simulink model "Fuel_Pump_V3_1_20201113_20KHz"  (R2019b)
settings: configuration reference "Configuration" (kept outside this file)
PreLoadFcn:
  | RTWConfigurationCB('preloadfcn', bdroot);
values from neighbouring files (symbols this model uses):
  MotorPara_Base_Frq = 666.0    [fuel_pump_V3_1_20201113_20kHz.sldd]
  MotorPara_Base_I = 50.0    [fuel_pump_V3_1_20201113_20kHz.sldd]
  MotorPara_Base_RPM = 12000.0    [fuel_pump_V3_1_20201113_20kHz.sldd]
  MotorPara_Base_V = 28.0    [fuel_pump_V3_1_20201113_20kHz.sldd]
  MotorPara_Ld = 1.287E-5    [fuel_pump_V3_1_20201113_20kHz.sldd]
  MotorPara_Lq = 2.052E-5    [fuel_pump_V3_1_20201113_20kHz.sldd]
  MotorPara_Ls = 8.3475E-5    [fuel_pump_V3_1_20201113_20kHz.sldd]
  MotorPara_P = 4.0    [fuel_pump_V3_1_20201113_20kHz.sldd]
  MotorPara_Rs = 0.01638    [fuel_pump_V3_1_20201113_20kHz.sldd]
  TPBRD_HALF = 1875.0    [fuel_pump_V3_1_20201113_20kHz.sldd]
  Ts_1kHz = 0.001    [fuel_pump_V3_1_20201113_20kHz.sldd]
  Ts_200Hz = 0.005    [fuel_pump_V3_1_20201113_20kHz.sldd]
  Ts_20KHz = 5.0E-5    [fuel_pump_V3_1_20201113_20kHz.sldd]
  Ts_40Hz = 0.025    [fuel_pump_V3_1_20201113_20kHz.sldd]
  Ts_50Hz = 0.02    [fuel_pump_V3_1_20201113_20kHz.sldd]
undefined symbols (not defined in the file or in its folder): DiscIntNeverNeededParam, Down, Up
libraries: c280xlib x22, c2833xlib x6, c2837xDlib x4, c28xdmclib x4, etargetslib x4, dspstat3 x2, c2000lib x1, idelinklib_common x1
(part 1 of 4)
settings Model: DataDictionary=fuel_pump_V3_1_20201113_20kHz.sldd  ExtModeTrigDuration=8  OrderedModelArguments=off  Creator=Downstream  LastModifiedBy=Downstream
settings ConfigSetRef: SourceName=Configuration

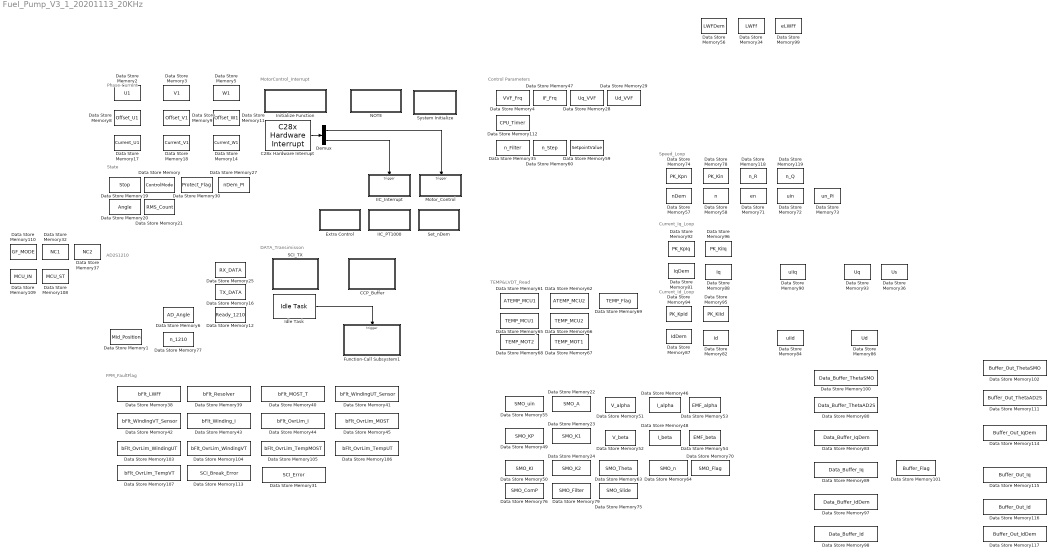
== system Fuel_Pump_V3_1_20201113_20KHz ==
  note: AD2S1210
  note: Phase-Current
  note: State
  note: DATA_Transimisson
  note: MotorControl_Interrupt
  note: Current_Id_Loop
  note: Current_Iq_Loop
  note: Control Parameters
  note: TEMP&LVDT_Read
  note: Speed_Loop
  note: FPM_FaultFlag
  C28x Hardware Interrupt : c2000lib/Scheduling/C28x Hardware Interrupt  irqnumbers=[1 8]  pienumbers=[6 1]  irqpriorities=[4 5]  irqpreempts=[0 0]  showinput=off  dspchiptype=C280X
      settings: SourceProductName=Embedded Coder Support Package for Texas Instruments C2000 Processors  SourceProductBaseCode=TIC2000
  CCP_Buffer : Subsystem  Priority=100  TreatAsAtomicUnit=on  SystemSampleTime=Ts_200Hz
  Data Store Memory : DataStoreMemory  DataStoreName=ControlMode  ReadBeforeWriteMsg=warning  WriteAfterWriteMsg=warning  WriteAfterReadMsg=warning  InitialValue=4  ShowAdditionalParam=off  OutDataTypeStr=uint16
      settings: RTWStateStorageClass=ExportedGlobal
  Data Store Memory1 : DataStoreMemory  DataStoreName=Mid_Position  ReadBeforeWriteMsg=warning  WriteAfterWriteMsg=warning  WriteAfterReadMsg=warning  ShowAdditionalParam=off  OutDataTypeStr=uint16
      settings: RTWStateStorageClass=ExportedGlobal
  Data Store Memory100 : DataStoreMemory  DataStoreName=Data_Buffer_ThetaSMO  ReadBeforeWriteMsg=warning  WriteAfterWriteMsg=warning  WriteAfterReadMsg=warning  InitialValue=zeros(1,1000)  ShowAdditionalParam=off  OutDataTypeStr=single
      settings: RTWStateStorageClass=ExportedGlobal
  Data Store Memory101 : DataStoreMemory  DataStoreName=Buffer_Flag  ReadBeforeWriteMsg=warning  WriteAfterWriteMsg=warning  WriteAfterReadMsg=warning  ShowAdditionalParam=off  OutDataTypeStr=uint16
      settings: RTWStateStorageClass=ExportedGlobal
  Data Store Memory102 : DataStoreMemory  DataStoreName=Buffer_Out_ThetaSMO  ReadBeforeWriteMsg=warning  WriteAfterWriteMsg=warning  WriteAfterReadMsg=warning  ShowAdditionalParam=off  OutDataTypeStr=single
      settings: RTWStateStorageClass=ExportedGlobal
  Data Store Memory103 : DataStoreMemory  DataStoreName=bFlt_OvrLim_WindingUT  ReadBeforeWriteMsg=warning  WriteAfterWriteMsg=warning  WriteAfterReadMsg=warning  ShowAdditionalParam=off  OutDataTypeStr=uint16
      settings: RTWStateStorageClass=ExportedGlobal
  Data Store Memory104 : DataStoreMemory  DataStoreName=bFlt_OvrLim_WindingVT  ReadBeforeWriteMsg=warning  WriteAfterWriteMsg=warning  WriteAfterReadMsg=warning  ShowAdditionalParam=off  OutDataTypeStr=uint16
      settings: RTWStateStorageClass=ExportedGlobal
  Data Store Memory105 : DataStoreMemory  DataStoreName=bFlt_OvrLim_TempMOST  ReadBeforeWriteMsg=warning  WriteAfterWriteMsg=warning  WriteAfterReadMsg=warning  ShowAdditionalParam=off  OutDataTypeStr=uint16
      settings: RTWStateStorageClass=ExportedGlobal
  Data Store Memory106 : DataStoreMemory  DataStoreName=bFlt_OvrLim_TempUT  ReadBeforeWriteMsg=warning  WriteAfterWriteMsg=warning  WriteAfterReadMsg=warning  ShowAdditionalParam=off  OutDataTypeStr=uint16
      settings: RTWStateStorageClass=ExportedGlobal
  Data Store Memory107 : DataStoreMemory  DataStoreName=bFlt_OvrLim_TempVT  ReadBeforeWriteMsg=warning  WriteAfterWriteMsg=warning  WriteAfterReadMsg=warning  ShowAdditionalParam=off  OutDataTypeStr=uint16
      settings: RTWStateStorageClass=ExportedGlobal
  Data Store Memory108 : DataStoreMemory  DataStoreName=MCU_ST  ReadBeforeWriteMsg=warning  WriteAfterWriteMsg=warning  WriteAfterReadMsg=warning  ShowAdditionalParam=off  OutDataTypeStr=uint16
      settings: RTWStateStorageClass=ExportedGlobal
  Data Store Memory109 : DataStoreMemory  DataStoreName=MCU_IN  ReadBeforeWriteMsg=warning  WriteAfterWriteMsg=warning  WriteAfterReadMsg=warning  ShowAdditionalParam=off  OutDataTypeStr=uint16
      settings: RTWStateStorageClass=ExportedGlobal
  Data Store Memory11 : DataStoreMemory  DataStoreName=Offset_W1  ReadBeforeWriteMsg=warning  WriteAfterWriteMsg=warning  WriteAfterReadMsg=warning  ShowAdditionalParam=off  OutDataTypeStr=uint16
      settings: RTWStateStorageClass=ExportedGlobal
  Data Store Memory110 : DataStoreMemory  DataStoreName=GF_MODE  ReadBeforeWriteMsg=warning  WriteAfterWriteMsg=warning  WriteAfterReadMsg=warning  ShowAdditionalParam=off  OutDataTypeStr=uint16
      settings: RTWStateStorageClass=ExportedGlobal
  Data Store Memory111 : DataStoreMemory  DataStoreName=Buffer_Out_ThetaAD2S  ReadBeforeWriteMsg=warning  WriteAfterWriteMsg=warning  WriteAfterReadMsg=warning  ShowAdditionalParam=off  OutDataTypeStr=single
      settings: RTWStateStorageClass=ExportedGlobal
  Data Store Memory112 : DataStoreMemory  DataStoreName=CPU_Timer  ReadBeforeWriteMsg=warning  WriteAfterWriteMsg=warning  WriteAfterReadMsg=warning  ShowAdditionalParam=off  OutDataTypeStr=uint32
      settings: RTWStateStorageClass=ExportedGlobal
  Data Store Memory113 : DataStoreMemory  DataStoreName=SCI_Break_Error  ReadBeforeWriteMsg=warning  WriteAfterWriteMsg=warning  WriteAfterReadMsg=warning  ShowAdditionalParam=off  OutDataTypeStr=uint16
      settings: RTWStateStorageClass=ExportedGlobal
  Data Store Memory114 : DataStoreMemory  DataStoreName=Buffer_Out_IqDem  ReadBeforeWriteMsg=warning  WriteAfterWriteMsg=warning  WriteAfterReadMsg=warning  ShowAdditionalParam=off  OutDataTypeStr=single
      settings: RTWStateStorageClass=ExportedGlobal
  Data Store Memory115 : DataStoreMemory  DataStoreName=Buffer_Out_Iq  ReadBeforeWriteMsg=warning  WriteAfterWriteMsg=warning  WriteAfterReadMsg=warning  ShowAdditionalParam=off  OutDataTypeStr=single
      settings: RTWStateStorageClass=ExportedGlobal
  Data Store Memory116 : DataStoreMemory  DataStoreName=Buffer_Out_Id  ReadBeforeWriteMsg=warning  WriteAfterWriteMsg=warning  WriteAfterReadMsg=warning  ShowAdditionalParam=off  OutDataTypeStr=single
      settings: RTWStateStorageClass=ExportedGlobal
  Data Store Memory117 : DataStoreMemory  DataStoreName=Buffer_Out_IdDem  ReadBeforeWriteMsg=warning  WriteAfterWriteMsg=warning  WriteAfterReadMsg=warning  ShowAdditionalParam=off  OutDataTypeStr=single
      settings: RTWStateStorageClass=ExportedGlobal
  Data Store Memory118 : DataStoreMemory  DataStoreName=n_R  ReadBeforeWriteMsg=warning  WriteAfterWriteMsg=warning  WriteAfterReadMsg=warning  ShowAdditionalParam=off  OutDataTypeStr=single
      settings: RTWStateStorageClass=ExportedGlobal
  Data Store Memory119 : DataStoreMemory  DataStoreName=n_Q  ReadBeforeWriteMsg=warning  WriteAfterWriteMsg=warning  WriteAfterReadMsg=warning  ShowAdditionalParam=off  OutDataTypeStr=single
      settings: RTWStateStorageClass=ExportedGlobal
  Data Store Memory12 : DataStoreMemory  DataStoreName=Ready_1210  ReadBeforeWriteMsg=warning  WriteAfterWriteMsg=warning  WriteAfterReadMsg=warning  ShowAdditionalParam=off  OutDataTypeStr=single
      settings: RTWStateStorageClass=ExportedGlobal
  Data Store Memory14 : DataStoreMemory  DataStoreName=Current_W1  ReadBeforeWriteMsg=warning  WriteAfterWriteMsg=warning  WriteAfterReadMsg=warning  ShowAdditionalParam=off  OutDataTypeStr=single
      settings: RTWStateStorageClass=ExportedGlobal
  Data Store Memory16 : DataStoreMemory  DataStoreName=TX_DATA  ReadBeforeWriteMsg=warning  WriteAfterWriteMsg=warning  WriteAfterReadMsg=warning  ShowAdditionalParam=off  OutDataTypeStr=uint16
      settings: RTWStateStorageClass=ExportedGlobal
  Data Store Memory17 : DataStoreMemory  DataStoreName=Current_U1  ReadBeforeWriteMsg=warning  WriteAfterWriteMsg=warning  WriteAfterReadMsg=warning  ShowAdditionalParam=off  OutDataTypeStr=single
      settings: RTWStateStorageClass=ExportedGlobal
  Data Store Memory18 : DataStoreMemory  DataStoreName=Current_V1  ReadBeforeWriteMsg=warning  WriteAfterWriteMsg=warning  WriteAfterReadMsg=warning  ShowAdditionalParam=off  OutDataTypeStr=single
      settings: RTWStateStorageClass=ExportedGlobal
  Data Store Memory19 : DataStoreMemory  DataStoreName=Stop  ReadBeforeWriteMsg=warning  WriteAfterWriteMsg=warning  WriteAfterReadMsg=warning  ShowAdditionalParam=off  OutDataTypeStr=uint16
      settings: RTWStateStorageClass=ExportedGlobal
  Data Store Memory2 : DataStoreMemory  DataStoreName=U1  ReadBeforeWriteMsg=warning  WriteAfterWriteMsg=warning  WriteAfterReadMsg=warning  ShowAdditionalParam=off  OutDataTypeStr=uint16
      settings: RTWStateStorageClass=ExportedGlobal
  Data Store Memory20 : DataStoreMemory  DataStoreName=Angle  ReadBeforeWriteMsg=warning  WriteAfterWriteMsg=warning  WriteAfterReadMsg=warning  ShowAdditionalParam=off  OutDataTypeStr=single
      settings: RTWStateStorageClass=ExportedGlobal
  Data Store Memory21 : DataStoreMemory  DataStoreName=RMS_Count  ReadBeforeWriteMsg=warning  WriteAfterWriteMsg=warning  WriteAfterReadMsg=warning  ShowAdditionalParam=off  OutDataTypeStr=uint16
      settings: RTWStateStorageClass=ExportedGlobal
  Data Store Memory22 : DataStoreMemory  DataStoreName=SMO_A  ReadBeforeWriteMsg=warning  WriteAfterWriteMsg=warning  WriteAfterReadMsg=warning  ShowAdditionalParam=off  OutDataTypeStr=single
      settings: RTWStateStorageClass=ExportedGlobal
  Data Store Memory23 : DataStoreMemory  DataStoreName=SMO_K1  ReadBeforeWriteMsg=warning  WriteAfterWriteMsg=warning  WriteAfterReadMsg=warning  ShowAdditionalParam=off  OutDataTypeStr=single
      settings: RTWStateStorageClass=ExportedGlobal
  Data Store Memory24 : DataStoreMemory  DataStoreName=SMO_K2  ReadBeforeWriteMsg=warning  WriteAfterWriteMsg=warning  WriteAfterReadMsg=warning  ShowAdditionalParam=off  OutDataTypeStr=single
      settings: RTWStateStorageClass=ExportedGlobal
  Data Store Memory25 : DataStoreMemory  DataStoreName=RX_DATA  ReadBeforeWriteMsg=warning  WriteAfterWriteMsg=warning  WriteAfterReadMsg=warning  ShowAdditionalParam=off  OutDataTypeStr=uint16
      settings: RTWStateStorageClass=ExportedGlobal
  Data Store Memory27 : DataStoreMemory  DataStoreName=nDem_PI  ReadBeforeWriteMsg=warning  WriteAfterWriteMsg=warning  WriteAfterReadMsg=warning  ShowAdditionalParam=off  OutDataTypeStr=single
      settings: RTWStateStorageClass=ExportedGlobal
  Data Store Memory28 : DataStoreMemory  DataStoreName=Uq_VVF  ReadBeforeWriteMsg=warning  WriteAfterWriteMsg=warning  WriteAfterReadMsg=warning  ShowAdditionalParam=off  OutDataTypeStr=single
      settings: RTWStateStorageClass=ExportedGlobal
  Data Store Memory29 : DataStoreMemory  DataStoreName=Ud_VVF  ReadBeforeWriteMsg=warning  WriteAfterWriteMsg=warning  WriteAfterReadMsg=warning  ShowAdditionalParam=off  OutDataTypeStr=single
      settings: RTWStateStorageClass=ExportedGlobal
  Data Store Memory3 : DataStoreMemory  DataStoreName=V1  ReadBeforeWriteMsg=warning  WriteAfterWriteMsg=warning  WriteAfterReadMsg=warning  ShowAdditionalParam=off  OutDataTypeStr=uint16
      settings: RTWStateStorageClass=ExportedGlobal
  Data Store Memory30 : DataStoreMemory  DataStoreName=Protect_Flag  ReadBeforeWriteMsg=warning  WriteAfterWriteMsg=warning  WriteAfterReadMsg=warning  ShowAdditionalParam=off  OutDataTypeStr=uint16
      settings: RTWStateStorageClass=ExportedGlobal
  Data Store Memory31 : DataStoreMemory  DataStoreName=SCI_Error  ReadBeforeWriteMsg=warning  WriteAfterWriteMsg=warning  WriteAfterReadMsg=warning  ShowAdditionalParam=off  OutDataTypeStr=uint16
      settings: RTWStateStorageClass=ExportedGlobal
  Data Store Memory32 : DataStoreMemory  DataStoreName=NC1  ReadBeforeWriteMsg=warning  WriteAfterWriteMsg=warning  WriteAfterReadMsg=warning  ShowAdditionalParam=off  OutDataTypeStr=uint16
      settings: RTWStateStorageClass=ExportedGlobal
  Data Store Memory34 : DataStoreMemory  DataStoreName=LWFf  ReadBeforeWriteMsg=warning  WriteAfterWriteMsg=warning  WriteAfterReadMsg=warning  ShowAdditionalParam=off  OutDataTypeStr=single
      settings: RTWStateStorageClass=ExportedGlobal
  Data Store Memory35 : DataStoreMemory  DataStoreName=n_Filter  ReadBeforeWriteMsg=warning  WriteAfterWriteMsg=warning  WriteAfterReadMsg=warning  InitialValue=2000  ShowAdditionalParam=off  OutDataTypeStr=single
      settings: RTWStateStorageClass=ExportedGlobal
  Data Store Memory36 : DataStoreMemory  DataStoreName=Us  ReadBeforeWriteMsg=warning  WriteAfterWriteMsg=warning  WriteAfterReadMsg=warning  ShowAdditionalParam=off  OutDataTypeStr=single
      settings: RTWStateStorageClass=ExportedGlobal
  Data Store Memory37 : DataStoreMemory  DataStoreName=NC2  ReadBeforeWriteMsg=warning  WriteAfterWriteMsg=warning  WriteAfterReadMsg=warning  ShowAdditionalParam=off  OutDataTypeStr=uint16
      settings: RTWStateStorageClass=ExportedGlobal
  Data Store Memory38 : DataStoreMemory  DataStoreName=bFlt_LWFf  ReadBeforeWriteMsg=warning  WriteAfterWriteMsg=warning  WriteAfterReadMsg=warning  ShowAdditionalParam=off  OutDataTypeStr=uint16
      settings: RTWStateStorageClass=ExportedGlobal
  Data Store Memory39 : DataStoreMemory  DataStoreName=bFlt_Resolver  ReadBeforeWriteMsg=warning  WriteAfterWriteMsg=warning  WriteAfterReadMsg=warning  ShowAdditionalParam=off  OutDataTypeStr=uint16
      settings: RTWStateStorageClass=ExportedGlobal
  Data Store Memory4 : DataStoreMemory  DataStoreName=VVF_Frq  ReadBeforeWriteMsg=warning  WriteAfterWriteMsg=warning  WriteAfterReadMsg=warning  ShowAdditionalParam=off  OutDataTypeStr=fixdt(1,32,29)
      settings: RTWStateStorageClass=ExportedGlobal
  Data Store Memory40 : DataStoreMemory  DataStoreName=bFlt_MOST_T  ReadBeforeWriteMsg=warning  WriteAfterWriteMsg=warning  WriteAfterReadMsg=warning  ShowAdditionalParam=off  OutDataTypeStr=uint16
      settings: RTWStateStorageClass=ExportedGlobal
  Data Store Memory41 : DataStoreMemory  DataStoreName=bFlt_WindingUT_Sensor  ReadBeforeWriteMsg=warning  WriteAfterWriteMsg=warning  WriteAfterReadMsg=warning  ShowAdditionalParam=off  OutDataTypeStr=uint16
      settings: RTWStateStorageClass=ExportedGlobal
  Data Store Memory42 : DataStoreMemory  DataStoreName=bFlt_WindingVT_Sensor  ReadBeforeWriteMsg=warning  WriteAfterWriteMsg=warning  WriteAfterReadMsg=warning  ShowAdditionalParam=off  OutDataTypeStr=uint16
      settings: RTWStateStorageClass=ExportedGlobal
  Data Store Memory43 : DataStoreMemory  DataStoreName=bFlt_Winding_I  ReadBeforeWriteMsg=warning  WriteAfterWriteMsg=warning  WriteAfterReadMsg=warning  ShowAdditionalParam=off  OutDataTypeStr=uint16
      settings: RTWStateStorageClass=ExportedGlobal
  Data Store Memory44 : DataStoreMemory  DataStoreName=bFlt_OvrLim_I  ReadBeforeWriteMsg=warning  WriteAfterWriteMsg=warning  WriteAfterReadMsg=warning  ShowAdditionalParam=off  OutDataTypeStr=uint16
      settings: RTWStateStorageClass=ExportedGlobal
  Data Store Memory45 : DataStoreMemory  DataStoreName=bFlt_OvrLim_MOST  ReadBeforeWriteMsg=warning  WriteAfterWriteMsg=warning  WriteAfterReadMsg=warning  ShowAdditionalParam=off  OutDataTypeStr=uint16
      settings: RTWStateStorageClass=ExportedGlobal
  Data Store Memory46 : DataStoreMemory  DataStoreName=I_alpha  ReadBeforeWriteMsg=warning  WriteAfterWriteMsg=warning  WriteAfterReadMsg=warning  ShowAdditionalParam=off  OutDataTypeStr=single
      settings: RTWStateStorageClass=ExportedGlobal
  Data Store Memory47 : DataStoreMemory  DataStoreName=IF_Frq  ReadBeforeWriteMsg=warning  WriteAfterWriteMsg=warning  WriteAfterReadMsg=warning  ShowAdditionalParam=off  OutDataTypeStr=fixdt(1,32,29)
      settings: RTWStateStorageClass=ExportedGlobal
  Data Store Memory48 : DataStoreMemory  DataStoreName=I_beta  ReadBeforeWriteMsg=warning  WriteAfterWriteMsg=warning  WriteAfterReadMsg=warning  ShowAdditionalParam=off  OutDataTypeStr=single
      settings: RTWStateStorageClass=ExportedGlobal
  Data Store Memory49 : DataStoreMemory  DataStoreName=SMO_KP  ReadBeforeWriteMsg=warning  WriteAfterWriteMsg=warning  WriteAfterReadMsg=warning  ShowAdditionalParam=off  OutDataTypeStr=single
      settings: RTWStateStorageClass=ExportedGlobal
  Data Store Memory5 : DataStoreMemory  DataStoreName=W1  ReadBeforeWriteMsg=warning  WriteAfterWriteMsg=warning  WriteAfterReadMsg=warning  ShowAdditionalParam=off  OutDataTypeStr=uint16
      settings: RTWStateStorageClass=ExportedGlobal
  Data Store Memory50 : DataStoreMemory  DataStoreName=SMO_KI  ReadBeforeWriteMsg=warning  WriteAfterWriteMsg=warning  WriteAfterReadMsg=warning  ShowAdditionalParam=off  OutDataTypeStr=single
      settings: RTWStateStorageClass=ExportedGlobal
  Data Store Memory51 : DataStoreMemory  DataStoreName=V_alpha  ReadBeforeWriteMsg=warning  WriteAfterWriteMsg=warning  WriteAfterReadMsg=warning  ShowAdditionalParam=off  OutDataTypeStr=single
      settings: RTWStateStorageClass=ExportedGlobal
  Data Store Memory52 : DataStoreMemory  DataStoreName=V_beta  ReadBeforeWriteMsg=warning  WriteAfterWriteMsg=warning  WriteAfterReadMsg=warning  ShowAdditionalParam=off  OutDataTypeStr=single
      settings: RTWStateStorageClass=ExportedGlobal
  Data Store Memory53 : DataStoreMemory  DataStoreName=EMF_alpha  ReadBeforeWriteMsg=warning  WriteAfterWriteMsg=warning  WriteAfterReadMsg=warning  ShowAdditionalParam=off  OutDataTypeStr=single
      settings: RTWStateStorageClass=ExportedGlobal
  Data Store Memory54 : DataStoreMemory  DataStoreName=EMF_beta  ReadBeforeWriteMsg=warning  WriteAfterWriteMsg=warning  WriteAfterReadMsg=warning  ShowAdditionalParam=off  OutDataTypeStr=single
      settings: RTWStateStorageClass=ExportedGlobal
  Data Store Memory55 : DataStoreMemory  DataStoreName=SMO_uin  ReadBeforeWriteMsg=warning  WriteAfterWriteMsg=warning  WriteAfterReadMsg=warning  ShowAdditionalParam=off  OutDataTypeStr=single
      settings: RTWStateStorageClass=ExportedGlobal
  Data Store Memory56 : DataStoreMemory  DataStoreName=LWFDem  ReadBeforeWriteMsg=warning  WriteAfterWriteMsg=warning  WriteAfterReadMsg=warning  ShowAdditionalParam=off  OutDataTypeStr=single
      settings: RTWStateStorageClass=ExportedGlobal
  Data Store Memory57 : DataStoreMemory  DataStoreName=nDem  ReadBeforeWriteMsg=warning  WriteAfterWriteMsg=warning  WriteAfterReadMsg=warning  ShowAdditionalParam=off  OutDataTypeStr=single
      settings: RTWStateStorageClass=ExportedGlobal
  Data Store Memory58 : DataStoreMemory  DataStoreName=n  ReadBeforeWriteMsg=warning  WriteAfterWriteMsg=warning  WriteAfterReadMsg=warning  ShowAdditionalParam=off  OutDataTypeStr=single
      settings: RTWStateStorageClass=ExportedGlobal
  Data Store Memory59 : DataStoreMemory  DataStoreName=SetpointValue  ReadBeforeWriteMsg=warning  WriteAfterWriteMsg=warning  WriteAfterReadMsg=warning  ShowAdditionalParam=off  OutDataTypeStr=single
      settings: RTWStateStorageClass=ExportedGlobal
  Data Store Memory6 : DataStoreMemory  DataStoreName=AD_Angle  ReadBeforeWriteMsg=warning  WriteAfterWriteMsg=warning  WriteAfterReadMsg=warning  ShowAdditionalParam=off  OutDataTypeStr=single
      settings: RTWStateStorageClass=ExportedGlobal
  Data Store Memory60 : DataStoreMemory  DataStoreName=n_Step  ReadBeforeWriteMsg=warning  WriteAfterWriteMsg=warning  WriteAfterReadMsg=warning  InitialValue=5/15000  ShowAdditionalParam=off  OutDataTypeStr=single
      settings: RTWStateStorageClass=ExportedGlobal
  Data Store Memory61 : DataStoreMemory  DataStoreName=ATEMP_MCU1  ReadBeforeWriteMsg=warning  WriteAfterWriteMsg=warning  WriteAfterReadMsg=warning  ShowAdditionalParam=off  OutDataTypeStr=uint16
      settings: RTWStateStorageClass=ExportedGlobal
  Data Store Memory62 : DataStoreMemory  DataStoreName=ATEMP_MCU2  ReadBeforeWriteMsg=warning  WriteAfterWriteMsg=warning  WriteAfterReadMsg=warning  ShowAdditionalParam=off  OutDataTypeStr=uint16
      settings: RTWStateStorageClass=ExportedGlobal
  Data Store Memory63 : DataStoreMemory  DataStoreName=SMO_Theta  ReadBeforeWriteMsg=warning  WriteAfterWriteMsg=warning  WriteAfterReadMsg=warning  ShowAdditionalParam=off  OutDataTypeStr=single
      settings: RTWStateStorageClass=ExportedGlobal
  Data Store Memory64 : DataStoreMemory  DataStoreName=SMO_n  ReadBeforeWriteMsg=warning  WriteAfterWriteMsg=warning  WriteAfterReadMsg=warning  ShowAdditionalParam=off  OutDataTypeStr=single
      settings: RTWStateStorageClass=ExportedGlobal
  Data Store Memory65 : DataStoreMemory  DataStoreName=TEMP_MCU1  ReadBeforeWriteMsg=warning  WriteAfterWriteMsg=warning  WriteAfterReadMsg=warning  ShowAdditionalParam=off  OutDataTypeStr=single
      settings: RTWStateStorageClass=ExportedGlobal
  Data Store Memory66 : DataStoreMemory  DataStoreName=TEMP_MCU2  ReadBeforeWriteMsg=warning  WriteAfterWriteMsg=warning  WriteAfterReadMsg=warning  ShowAdditionalParam=off  OutDataTypeStr=single
      settings: RTWStateStorageClass=ExportedGlobal
  Data Store Memory67 : DataStoreMemory  DataStoreName=TEMP_MOT1  ReadBeforeWriteMsg=warning  WriteAfterWriteMsg=warning  WriteAfterReadMsg=warning  ShowAdditionalParam=off  OutDataTypeStr=single
      settings: RTWStateStorageClass=ExportedGlobal
  Data Store Memory68 : DataStoreMemory  DataStoreName=TEMP_MOT2  ReadBeforeWriteMsg=warning  WriteAfterWriteMsg=warning  WriteAfterReadMsg=warning  ShowAdditionalParam=off  OutDataTypeStr=single
      settings: RTWStateStorageClass=ExportedGlobal
  Data Store Memory69 : DataStoreMemory  DataStoreName=TEMP_Flag  ReadBeforeWriteMsg=warning  WriteAfterWriteMsg=warning  WriteAfterReadMsg=warning  ShowAdditionalParam=off  OutDataTypeStr=uint16
      settings: RTWStateStorageClass=ExportedGlobal
  Data Store Memory70 : DataStoreMemory  DataStoreName=SMO_Flag  ReadBeforeWriteMsg=warning  WriteAfterWriteMsg=warning  WriteAfterReadMsg=warning  ShowAdditionalParam=off  OutDataTypeStr=uint16
      settings: RTWStateStorageClass=ExportedGlobal
  Data Store Memory71 : DataStoreMemory  DataStoreName=en  ReadBeforeWriteMsg=warning  WriteAfterWriteMsg=warning  WriteAfterReadMsg=warning  ShowAdditionalParam=off  OutDataTypeStr=single
      settings: RTWStateStorageClass=ExportedGlobal
  Data Store Memory72 : DataStoreMemory  DataStoreName=uin  ReadBeforeWriteMsg=warning  WriteAfterWriteMsg=warning  WriteAfterReadMsg=warning  ShowAdditionalParam=off  OutDataTypeStr=single
      settings: RTWStateStorageClass=ExportedGlobal
  Data Store Memory73 : DataStoreMemory  DataStoreName=un_PI  ReadBeforeWriteMsg=warning  WriteAfterWriteMsg=warning  WriteAfterReadMsg=warning  ShowAdditionalParam=off  OutDataTypeStr=single
      settings: RTWStateStorageClass=ExportedGlobal
  Data Store Memory74 : DataStoreMemory  DataStoreName=PK_Kpn  ReadBeforeWriteMsg=warning  WriteAfterWriteMsg=warning  WriteAfterReadMsg=warning  ShowAdditionalParam=off  OutDataTypeStr=single
      settings: RTWStateStorageClass=ExportedGlobal
  Data Store Memory75 : DataStoreMemory  DataStoreName=SMO_Slide  ReadBeforeWriteMsg=warning  WriteAfterWriteMsg=warning  WriteAfterReadMsg=warning  ShowAdditionalParam=off  OutDataTypeStr=single
      settings: RTWStateStorageClass=ExportedGlobal
  Data Store Memory76 : DataStoreMemory  DataStoreName=SMO_ComP  ReadBeforeWriteMsg=warning  WriteAfterWriteMsg=warning  WriteAfterReadMsg=warning  ShowAdditionalParam=off  OutDataTypeStr=single
      settings: RTWStateStorageClass=ExportedGlobal
  Data Store Memory77 : DataStoreMemory  DataStoreName=n_1210  ReadBeforeWriteMsg=warning  WriteAfterWriteMsg=warning  WriteAfterReadMsg=warning  ShowAdditionalParam=off  OutDataTypeStr=single
      settings: RTWStateStorageClass=ExportedGlobal
  Data Store Memory78 : DataStoreMemory  DataStoreName=PK_Kin  ReadBeforeWriteMsg=warning  WriteAfterWriteMsg=warning  WriteAfterReadMsg=warning  ShowAdditionalParam=off  OutDataTypeStr=single
      settings: RTWStateStorageClass=ExportedGlobal
  Data Store Memory79 : DataStoreMemory  DataStoreName=SMO_Filter  ReadBeforeWriteMsg=warning  WriteAfterWriteMsg=warning  WriteAfterReadMsg=warning  ShowAdditionalParam=off  OutDataTypeStr=single
      settings: RTWStateStorageClass=ExportedGlobal
  Data Store Memory8 : DataStoreMemory  DataStoreName=Offset_U1  ReadBeforeWriteMsg=warning  WriteAfterWriteMsg=warning  WriteAfterReadMsg=warning  ShowAdditionalParam=off  OutDataTypeStr=uint16
      settings: RTWStateStorageClass=ExportedGlobal
  Data Store Memory80 : DataStoreMemory  DataStoreName=Data_Buffer_ThetaAD2S  ReadBeforeWriteMsg=warning  WriteAfterWriteMsg=warning  WriteAfterReadMsg=warning  InitialValue=zeros(1,1000)  ShowAdditionalParam=off  OutDataTypeStr=single
      settings: RTWStateStorageClass=ExportedGlobal
  Data Store Memory81 : DataStoreMemory  DataStoreName=IqDem  ReadBeforeWriteMsg=warning  WriteAfterWriteMsg=warning  WriteAfterReadMsg=warning  ShowAdditionalParam=off  OutDataTypeStr=single
      settings: RTWStateStorageClass=ExportedGlobal
  Data Store Memory82 : DataStoreMemory  DataStoreName=Id  ReadBeforeWriteMsg=warning  WriteAfterWriteMsg=warning  WriteAfterReadMsg=warning  ShowAdditionalParam=off  OutDataTypeStr=single
      settings: RTWStateStorageClass=ExportedGlobal
  Data Store Memory83 : DataStoreMemory  DataStoreName=Data_Buffer_IqDem  ReadBeforeWriteMsg=warning  WriteAfterWriteMsg=warning  WriteAfterReadMsg=warning  InitialValue=zeros(1,1000)  ShowAdditionalParam=off  OutDataTypeStr=single
      settings: RTWStateStorageClass=ExportedGlobal
  Data Store Memory84 : DataStoreMemory  DataStoreName=uiId  ReadBeforeWriteMsg=warning  WriteAfterWriteMsg=warning  WriteAfterReadMsg=warning  ShowAdditionalParam=off  OutDataTypeStr=single
      settings: RTWStateStorageClass=ExportedGlobal
  Data Store Memory86 : DataStoreMemory  DataStoreName=Ud  ReadBeforeWriteMsg=warning  WriteAfterWriteMsg=warning  WriteAfterReadMsg=warning  ShowAdditionalParam=off  OutDataTypeStr=single
      settings: RTWStateStorageClass=ExportedGlobal
  Data Store Memory87 : DataStoreMemory  DataStoreName=IdDem  ReadBeforeWriteMsg=warning  WriteAfterWriteMsg=warning  WriteAfterReadMsg=warning  ShowAdditionalParam=off  OutDataTypeStr=single
      settings: RTWStateStorageClass=ExportedGlobal
  Data Store Memory88 : DataStoreMemory  DataStoreName=Iq  ReadBeforeWriteMsg=warning  WriteAfterWriteMsg=warning  WriteAfterReadMsg=warning  ShowAdditionalParam=off  OutDataTypeStr=single
      settings: RTWStateStorageClass=ExportedGlobal
  Data Store Memory89 : DataStoreMemory  DataStoreName=Data_Buffer_Iq  ReadBeforeWriteMsg=warning  WriteAfterWriteMsg=warning  WriteAfterReadMsg=warning  InitialValue=zeros(1,1000)  ShowAdditionalParam=off  OutDataTypeStr=single
      settings: RTWStateStorageClass=ExportedGlobal
  Data Store Memory9 : DataStoreMemory  DataStoreName=Offset_V1  ReadBeforeWriteMsg=warning  WriteAfterWriteMsg=warning  WriteAfterReadMsg=warning  ShowAdditionalParam=off  OutDataTypeStr=uint16
      settings: RTWStateStorageClass=ExportedGlobal
  Data Store Memory90 : DataStoreMemory  DataStoreName=uiIq  ReadBeforeWriteMsg=warning  WriteAfterWriteMsg=warning  WriteAfterReadMsg=warning  ShowAdditionalParam=off  OutDataTypeStr=single
      settings: RTWStateStorageClass=ExportedGlobal
  Data Store Memory92 : DataStoreMemory  DataStoreName=PK_KpIq  ReadBeforeWriteMsg=warning  WriteAfterWriteMsg=warning  WriteAfterReadMsg=warning  ShowAdditionalParam=off  OutDataTypeStr=single
      settings: RTWStateStorageClass=ExportedGlobal
  Data Store Memory93 : DataStoreMemory  DataStoreName=Uq  ReadBeforeWriteMsg=warning  WriteAfterWriteMsg=warning  WriteAfterReadMsg=warning  ShowAdditionalParam=off  OutDataTypeStr=single
      settings: RTWStateStorageClass=ExportedGlobal
  Data Store Memory94 : DataStoreMemory  DataStoreName=PK_KpId  ReadBeforeWriteMsg=warning  WriteAfterWriteMsg=warning  WriteAfterReadMsg=warning  ShowAdditionalParam=off  OutDataTypeStr=single
      settings: RTWStateStorageClass=ExportedGlobal
  Data Store Memory95 : DataStoreMemory  DataStoreName=PK_KiId  ReadBeforeWriteMsg=warning  WriteAfterWriteMsg=warning  WriteAfterReadMsg=warning  ShowAdditionalParam=off  OutDataTypeStr=single
      settings: RTWStateStorageClass=ExportedGlobal
  Data Store Memory96 : DataStoreMemory  DataStoreName=PK_KiIq  ReadBeforeWriteMsg=warning  WriteAfterWriteMsg=warning  WriteAfterReadMsg=warning  ShowAdditionalParam=off  OutDataTypeStr=single
      settings: RTWStateStorageClass=ExportedGlobal
  Data Store Memory97 : DataStoreMemory  DataStoreName=Data_Buffer_IdDem  ReadBeforeWriteMsg=warning  WriteAfterWriteMsg=warning  WriteAfterReadMsg=warning  InitialValue=zeros(1,1000)  ShowAdditionalParam=off  OutDataTypeStr=single
      settings: RTWStateStorageClass=ExportedGlobal
  Data Store Memory98 : DataStoreMemory  DataStoreName=Data_Buffer_Id  ReadBeforeWriteMsg=warning  WriteAfterWriteMsg=warning  WriteAfterReadMsg=warning  InitialValue=zeros(1,1000)  ShowAdditionalParam=off  OutDataTypeStr=single
      settings: RTWStateStorageClass=ExportedGlobal
  Data Store Memory99 : DataStoreMemory  DataStoreName=eLWFf  ReadBeforeWriteMsg=warning  WriteAfterWriteMsg=warning  WriteAfterReadMsg=warning  ShowAdditionalParam=off  OutDataTypeStr=single
      settings: RTWStateStorageClass=ExportedGlobal
  Demux : Demux  Outputs=2
  "Extra Control " : Subsystem
  Function-Call Subsystem1 : Subsystem  TreatAsAtomicUnit=on
  "IIC_Interrupt " : Subsystem
      settings: RTWMemSecFuncInitTerm=code_ramfuncs
  IIC_PT1000 : Subsystem  TreatAsAtomicUnit=on  SystemSampleTime=Ts_50Hz
  Idle Task : idelinklib_common/Idle Task  tasknumbers=[1]  taskpriorities=100017  taskpreempts=[1]  showinput=off  simPriority=0
      settings: SourceProductName=MATLAB Coder  SourceProductBaseCode=ME
  Initialize Function : Subsystem  TreatAsAtomicUnit=on
  Motor_Control : Subsystem  TreatAsAtomicUnit=on
      settings: RTWSystemCode=Nonreusable function  RTWMemSecFuncInitTerm=code_ramfuncs
  NOTE : Subsystem
  SCI_TX : Subsystem  Priority=100
  Set_nDem : Subsystem  TreatAsAtomicUnit=on  SystemSampleTime=1e-3
      settings: RTWSystemCode=Nonreusable function  RTWMemSecFuncInitTerm=code_ramfuncs
  System Initialize : Subsystem  mask(System Initialize){ShowInLibBrowser=0}
      mask prompts: ShowInLibBrowser "Simulink:masks:CustCodeMaskParam1_MP"
      settings: CopyFcn=cccopyfcn(gcb)  OpenFcn=ccopenfcn('System Initialize Function')
      mask Help: eval('feval(''rtwprivate'',''rtwhelpview'',''rtw_sys_initialize_block'')');
      mask Display: disp('System\nInitialize');
  wires:
  Demux/2 -> "IIC_Interrupt "/Trigger
  Demux/1 -> Motor_Control/Trigger
  Idle Task/1 -> Function-Call Subsystem1/Trigger
  C28x Hardware Interrupt/1 -> Demux/1

== system Fuel_Pump_V3_1_20201113_20KHz/CCP_Buffer ==
  MATLAB Function : MATLAB Function  TreatAsAtomicUnit=on

== system Fuel_Pump_V3_1_20201113_20KHz/Extra Control  ==
  Data Store Read : DataStoreRead  Commented=on  DataStoreName=MCU_IN
  Data Store Write10 : DataStoreWrite  DataStoreName=MCU_ST
  Data Store Write7 : DataStoreWrite  DataStoreName=GF_MODE
  Data Store Write8 : DataStoreWrite  DataStoreName=NC1
  Data Store Write9 : DataStoreWrite  DataStoreName=NC2
  Demux : Demux  Outputs=3
  Digital Input : c2833xlib/Digital Input  GPIO_Number=GPIO48~GPIO55  GPIO_Bit0=off  GPIO_Bit1=off  GPIO_Bit2=off  GPIO_Bit3=off  GPIO_Bit4=off  GPIO_Bit5=on  GPIO_Bit6=on  GPIO_Bit7=on  sampleTime=Ts_1kHz  dataType=auto  GPIO_Bit0_Qualification=Sync to SYSCLKOUT  GPIO_Bit1_Qualification=Sync to SYSCLKOUT  GPIO_Bit2_Qualification=Sync to SYSCLKOUT  GPIO_Bit3_Qualification=Sync to SYSCLKOUT  GPIO_Bit4_Qualification=Sync to SYSCLKOUT  GPIO_Bit5_Qualification=Sync to SYSCLKOUT  GPIO_Bit6_Qualification=Sync to SYSCLKOUT  GPIO_Bit7_Qualification=Sync to SYSCLKOUT  Qualification_Period=-1
      settings: SourceProductName=Embedded Coder Support Package for Texas Instruments C2000 Processors  SourceProductBaseCode=TIC2000
  Digital Input1 : c2833xlib/Digital Input  GPIO_Number=GPIO56~GPIO63  GPIO_Bit0=on  GPIO_Bit1=off  GPIO_Bit2=off  GPIO_Bit3=off  GPIO_Bit4=off  GPIO_Bit5=off  GPIO_Bit6=off  GPIO_Bit7=off  sampleTime=Ts_1kHz  dataType=auto  GPIO_Bit0_Qualification=Sync to SYSCLKOUT  GPIO_Bit1_Qualification=Sync to SYSCLKOUT  GPIO_Bit2_Qualification=Sync to SYSCLKOUT  GPIO_Bit3_Qualification=Sync to SYSCLKOUT  GPIO_Bit4_Qualification=Sync to SYSCLKOUT  GPIO_Bit5_Qualification=Sync to SYSCLKOUT  GPIO_Bit6_Qualification=Sync to SYSCLKOUT  GPIO_Bit7_Qualification=Sync to SYSCLKOUT  Qualification_Period=-1
      settings: SourceProductName=Embedded Coder Support Package for Texas Instruments C2000 Processors  SourceProductBaseCode=TIC2000
  Digital Output : c2833xlib/Digital Output  Commented=on  GPIO_Number=GPIO48~GPIO55  GPIO_Bit0=off  GPIO_BIT0_Toggle=off  GPIO_Bit1=off  GPIO_BIT1_Toggle=off  GPIO_Bit2=off  GPIO_BIT2_Toggle=off  GPIO_Bit3=off  GPIO_BIT3_Toggle=off  GPIO_Bit4=on  GPIO_BIT4_Toggle=off  GPIO_Bit5=off  GPIO_BIT5_Toggle=off  GPIO_Bit6=off  GPIO_BIT6_Toggle=off  GPIO_Bit7=off  GPIO_BIT7_Toggle=off
      settings: SourceProductName=Embedded Coder Support Package for Texas Instruments C2000 Processors  SourceProductBaseCode=TIC2000
  wires:
  Demux/1 -> Data Store Write10/1
  Data Store Read/1 -> Digital Output/1
  Digital Input/1 -> Demux/1
  Demux/2 -> Data Store Write7/1
  Digital Input1/1 -> Data Store Write9/1
  Demux/3 -> Data Store Write8/1

== system Fuel_Pump_V3_1_20201113_20KHz/Function-Call Subsystem1 ==
  function : TriggerPort  TriggerType=function-call  VariantControl=Variant
  CAN Calibration Protocol : c280xlib/CAN Calibration Protocol  CCP_STATION_ID=hex2dec('1')  module=eCAN_A  ccp_cro_id=hex2dec('6FA')  ccp_cro_message_type=Standard (11-bit identifier)  ccp_return_id=hex2dec('6FB')  ccp_return_message_type=Standard (11-bit identifier)  TOTAL_NUM_ODTS=8  cro_sample_time=-1
      settings: SourceProductName=Embedded Coder Support Package for Texas Instruments C2000 Processors  SourceProductBaseCode=TIC2000
  Data Store Read : DataStoreRead  DataStoreName=ATEMP_MCU1
  Data Store Read1 : DataStoreRead  DataStoreName=ATEMP_MCU2
  Data Store Write : DataStoreWrite  DataStoreName=TEMP_MCU2
  Data Store Write1 : DataStoreWrite  DataStoreName=TEMP_MCU1
  Moving Average : dspstat3/Moving Average  Method=Sliding window  ForgettingFactorPort=off  SpecifyWindowLength=on  WindowLength=40  ForgettingFactor=0.9  SimulateUsing=Code generation
  Moving Average1 : dspstat3/Moving Average  Method=Sliding window  ForgettingFactorPort=off  SpecifyWindowLength=on  WindowLength=40  ForgettingFactor=0.9  SimulateUsing=Code generation
  READ Temp : MATLAB Function  TreatAsAtomicUnit=on
  READ Temp1 : MATLAB Function  TreatAsAtomicUnit=on
  wires:
  Data Store Read/1 -> READ Temp/1(AD)
  Data Store Read1/1 -> READ Temp1/1(AD)
  READ Temp/1(TEMP) -> Moving Average/1
  READ Temp1/1(TEMP) -> Moving Average1/1
  Moving Average/1 -> Data Store Write1/1
  Moving Average1/1 -> Data Store Write/1

== system Fuel_Pump_V3_1_20201113_20KHz/IIC_Interrupt  ==
  function : TriggerPort  TriggerType=function-call  VariantControl=Variant
  MATLAB Function : MATLAB Function  TreatAsAtomicUnit=on
  Subsystem : Subsystem
  Subsystem1 : Subsystem
  wires:
  MATLAB Function/1(TEMP1()) -> Subsystem/Trigger
  MATLAB Function/2(TEMP2()) -> Subsystem1/Trigger

== system Fuel_Pump_V3_1_20201113_20KHz/IIC_PT1000 ==
  MATLAB Function : MATLAB Function  TreatAsAtomicUnit=on  SystemSampleTime=Ts_50Hz
  Subsystem4 : Subsystem
  Subsystem5 : Subsystem
  wires:
  MATLAB Function/2(TEMP2()) -> Subsystem5/Trigger
  MATLAB Function/1(TEMP1()) -> Subsystem4/Trigger

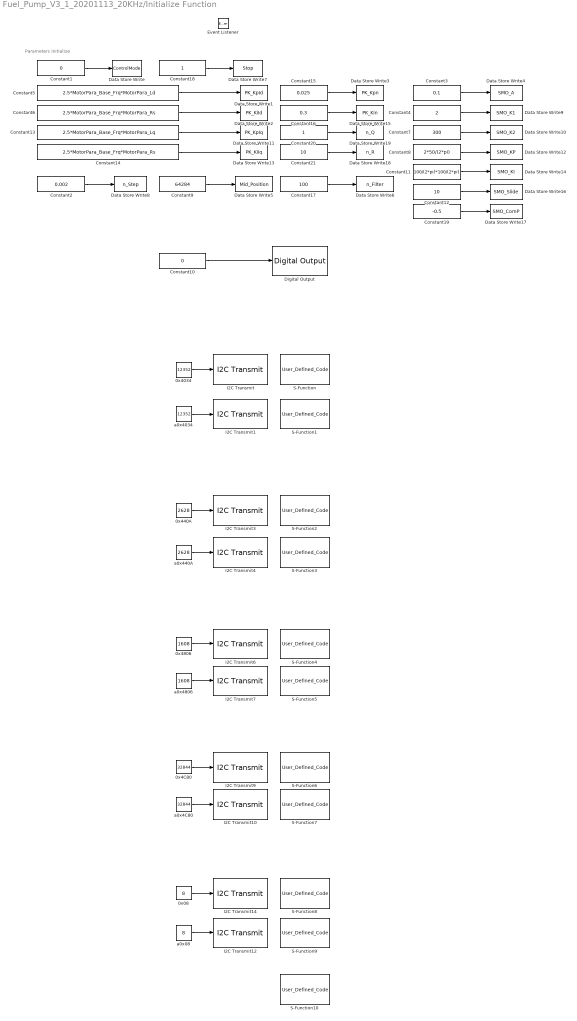
== system Fuel_Pump_V3_1_20201113_20KHz/Initialize Function ==
  note: Parameters Initialize
  0x08 : Constant  Priority=25  Value=8  OutDataTypeStr=uint8
  0x4034 : Constant  Priority=1  Value=12352  OutDataTypeStr=uint16
  0x440A : Constant  Priority=7  Value=2628  OutDataTypeStr=uint16
  0x4806 : Constant  Priority=13  Value=1608  OutDataTypeStr=uint16
  0x4C80 : Constant  Priority=19  Value=32844  OutDataTypeStr=uint16
  Constant1 : Constant  Value=0  OutDataTypeStr=uint16
  Constant10 : Constant  Value=0  OutDataTypeStr=uint16
  Constant11 : Constant  Value=100/(2*pi)*100/(2*pi)  OutDataTypeStr=single
  Constant12 : Constant  Value=10  OutDataTypeStr=single
  Constant13 : Constant  Value=2.5*MotorPara_Base_Frq*MotorPara_Lq  OutDataTypeStr=single
  Constant14 : Constant  Value=2.5*MotorPara_Base_Frq*MotorPara_Rs  OutDataTypeStr=single
  Constant15 : Constant  Value=0.025  OutDataTypeStr=single
  Constant16 : Constant  Value=0.3  OutDataTypeStr=single
  Constant17 : Constant  Value=100  OutDataTypeStr=single
  Constant18 : Constant  OutDataTypeStr=uint16
  Constant19 : Constant  Value=-0.5  OutDataTypeStr=single
  Constant2 : Constant  Value=0.002  OutDataTypeStr=single
  Constant20 : Constant  OutDataTypeStr=single  SampleTime=-1
  Constant21 : Constant  Value=10  OutDataTypeStr=single  SampleTime=-1
  Constant3 : Constant  Value=0.1  OutDataTypeStr=single
  Constant4 : Constant  Value=2  OutDataTypeStr=single
  Constant5 : Constant  Value=2.5*MotorPara_Base_Frq*MotorPara_Ld  OutDataTypeStr=single
  Constant6 : Constant  Value=2.5*MotorPara_Base_Frq*MotorPara_Rs  OutDataTypeStr=single
  Constant7 : Constant  Value=300  OutDataTypeStr=single
  Constant8 : Constant  Value=2*50/(2*pi)  OutDataTypeStr=single
  Constant9 : Constant  Value=64284  OutDataTypeStr=uint16
  Data Store Write : DataStoreWrite  DataStoreName=ControlMode
  Data Store Write1 : DataStoreWrite  DataStoreName=PK_KpId
  Data Store Write10 : DataStoreWrite  DataStoreName=SMO_K2
  Data Store Write11 : DataStoreWrite  DataStoreName=PK_KpIq
  Data Store Write12 : DataStoreWrite  DataStoreName=SMO_KP
  Data Store Write13 : DataStoreWrite  DataStoreName=PK_KiIq
  Data Store Write14 : DataStoreWrite  DataStoreName=SMO_KI
  Data Store Write15 : DataStoreWrite  DataStoreName=PK_Kin
  Data Store Write16 : DataStoreWrite  DataStoreName=SMO_Slide
  Data Store Write17 : DataStoreWrite  DataStoreName=SMO_ComP
  Data Store Write18 : DataStoreWrite  DataStoreName=n_R
  Data Store Write19 : DataStoreWrite  DataStoreName=n_Q
  Data Store Write2 : DataStoreWrite  DataStoreName=PK_KiId
  Data Store Write3 : DataStoreWrite  DataStoreName=PK_Kpn
  Data Store Write4 : DataStoreWrite  DataStoreName=SMO_A
  Data Store Write5 : DataStoreWrite  DataStoreName=Mid_Position
  Data Store Write6 : DataStoreWrite  DataStoreName=n_Filter
  Data Store Write7 : DataStoreWrite  DataStoreName=Stop
  Data Store Write8 : DataStoreWrite  DataStoreName=n_Step
  Data Store Write9 : DataStoreWrite  DataStoreName=SMO_K1
  Digital Output : c2833xlib/Digital Output  GPIO_Number=GPIO48~GPIO55  GPIO_Bit0=off  GPIO_BIT0_Toggle=off  GPIO_Bit1=off  GPIO_BIT1_Toggle=off  GPIO_Bit2=off  GPIO_BIT2_Toggle=off  GPIO_Bit3=off  GPIO_BIT3_Toggle=off  GPIO_Bit4=on  GPIO_BIT4_Toggle=off  GPIO_Bit5=off  GPIO_BIT5_Toggle=off  GPIO_Bit6=off  GPIO_BIT6_Toggle=off  GPIO_Bit7=off  GPIO_BIT7_Toggle=off
      settings: SourceProductName=Embedded Coder Support Package for Texas Instruments C2000 Processors  SourceProductBaseCode=TIC2000
  Event Listener : EventListener  DisableCoverage=on  EventName=reset
  I2C Transmit{,3,6,9,14} (5 alike) : c280xlib/I2C Transmit  selectModule=I2C_A  addrFormat=7-Bit addressing  saSource=Specify via dialog  SAR=64  bitCount=8  STP=on  RM=off  STR=off
      settings: SourceProductName=Embedded Coder Support Package for Texas Instruments C2000 Processors  SourceProductBaseCode=TIC2000
  I2C Transmit{1,4,7,10,12} (5 alike) : c280xlib/I2C Transmit  selectModule=I2C_A  addrFormat=7-Bit addressing  saSource=Specify via dialog  SAR=65  bitCount=8  STP=on  RM=off  STR=off
      settings: SourceProductName=Embedded Coder Support Package for Texas Instruments C2000 Processors  SourceProductBaseCode=TIC2000
  S-Function : S-Function  Priority=3  FunctionName=User_Defined_Code  Parameters=code  SFunctionDeploymentMode=off  EnableBusSupport=off  mask{code=DELAY_US(800L);}
  S-Function1 : S-Function  Priority=6  FunctionName=User_Defined_Code  Parameters=code  SFunctionDeploymentMode=off  EnableBusSupport=off  mask{code=DELAY_US(800L);}
  S-Function10 : S-Function  Priority=32  FunctionName=User_Defined_Code  Parameters=code  SFunctionDeploymentMode=off  EnableBusSupport=off  mask{code=DELAY_US(8000L);}
  S-Function2 : S-Function  Priority=9  FunctionName=User_Defined_Code  Parameters=code  SFunctionDeploymentMode=off  EnableBusSupport=off  mask{code=DELAY_US(800L);}
  S-Function3 : S-Function  Priority=12  FunctionName=User_Defined_Code  Parameters=code  SFunctionDeploymentMode=off  EnableBusSupport=off  mask{code=DELAY_US(800L);}
  S-Function4 : S-Function  Priority=15  FunctionName=User_Defined_Code  Parameters=code  SFunctionDeploymentMode=off  EnableBusSupport=off  mask{code=DELAY_US(800L);}
  S-Function5 : S-Function  Priority=18  FunctionName=User_Defined_Code  Parameters=code  SFunctionDeploymentMode=off  EnableBusSupport=off  mask{code=DELAY_US(800L);}
  S-Function6 : S-Function  Priority=21  FunctionName=User_Defined_Code  Parameters=code  SFunctionDeploymentMode=off  EnableBusSupport=off  mask{code=DELAY_US(800L);}
  S-Function7 : S-Function  Priority=24  FunctionName=User_Defined_Code  Parameters=code  SFunctionDeploymentMode=off  EnableBusSupport=off  mask{code=DELAY_US(800L);}
  S-Function8 : S-Function  Priority=27  FunctionName=User_Defined_Code  Parameters=code  SFunctionDeploymentMode=off  EnableBusSupport=off  mask{code=DELAY_US(800L);}
  S-Function9 : S-Function  Priority=30  FunctionName=User_Defined_Code  Parameters=code  SFunctionDeploymentMode=off  EnableBusSupport=off  mask{code=DELAY_US(800L);}
  a0x08 : Constant  Priority=28  Value=8  OutDataTypeStr=uint8
  a0x4034 : Constant  Priority=4  Value=12352  OutDataTypeStr=uint16
  a0x440A : Constant  Priority=10  Value=2628  OutDataTypeStr=uint16
  a0x4806 : Constant  Priority=16  Value=1608  OutDataTypeStr=uint16
  a0x4C80 : Constant  Priority=22  Value=32844  OutDataTypeStr=uint16
  wires:
  Constant1/1 -> Data Store Write/1
  Constant5/1 -> Data Store Write1/1
  Constant6/1 -> Data Store Write2/1
  Constant2/1 -> Data Store Write8/1
  Constant14/1 -> Data Store Write13/1
  Constant13/1 -> Data Store Write11/1
  Constant15/1 -> Data Store Write3/1
  Constant16/1 -> Data Store Write15/1
  0x4C80/1 -> I2C Transmit9/1
  0x4806/1 -> I2C Transmit6/1
  a0x4034/1 -> I2C Transmit1/1
  0x440A/1 -> I2C Transmit3/1
  a0x08/1 -> I2C Transmit12/1
  a0x4C80/1 -> I2C Transmit10/1
  0x4034/1 -> I2C Transmit/1
  a0x4806/1 -> I2C Transmit7/1
  0x08/1 -> I2C Transmit14/1
  a0x440A/1 -> I2C Transmit4/1
  Constant9/1 -> Data Store Write5/1
  Constant10/1 -> Digital Output/1
  Constant17/1 -> Data Store Write6/1
  Constant18/1 -> Data Store Write7/1
  Constant3/1 -> Data Store Write4/1
  Constant4/1 -> Data Store Write9/1
  Constant7/1 -> Data Store Write10/1
  Constant8/1 -> Data Store Write12/1
  Constant11/1 -> Data Store Write14/1
  Constant12/1 -> Data Store Write16/1
  Constant19/1 -> Data Store Write17/1
  Constant20/1 -> Data Store Write19/1
  Constant21/1 -> Data Store Write18/1

== system Fuel_Pump_V3_1_20201113_20KHz/Motor_Control ==
  function : TriggerPort  TriggerType=function-call  VariantControl=Variant
  ADC : c280xlib/ADC  Priority=3  useModule=A  useMode=Sequential  sourceSOC=ePWMxA  sourceSOC1=ePWMxA  sourceSOC2=ePWMxB  xint2_ADCSOC=31  Ts=-1  dType=uint16  postInterrupt=on  numConversionsSingle=5  numConversionsDouble=1  conv0=ADCINA0  conv1=ADCINA1  conv2=ADCINA2  conv3=ADCINA3  conv4=ADCINA4  conv5=ADCINA5  conv6=ADCINA6  conv7=ADCINA7  conv8=ADCINB0  conv9=ADCINB1  conv10=ADCINB2  conv11=ADCINB3  conv12=ADCINB4  conv13=ADCINB5  conv14=ADCINB6  conv15=ADCINB7  convAB0=ADCINA0 and ADCINB0  convAB1=ADCINA1 and ADCINB1  convAB2=ADCINA2 and ADCINB2  convAB3=ADCINA3 and ADCINB3  convAB4=ADCINA4 and ADCINB4  convAB5=ADCINA5 and ADCINB5  convAB6=ADCINA6 and ADCINB6  convAB7=ADCINA7 and ADCINB7  convA0=ADCINA0  convA1=ADCINA1  convA2=ADCINA2  convA3=ADCINA3  convA4=ADCINA4  convA5=ADCINA5  convA6=ADCINA6  convA7=ADCINA7  convB0=ADCINB0  convB1=ADCINB1  convB2=ADCINB2  convB3=ADCINB3  convB4=ADCINB4  convB5=ADCINB5  convB6=ADCINB6  convB7=ADCINB7  c28xmultiPort=off  endma=off  chdma=1
      settings: SourceProductName=Embedded Coder Support Package for Texas Instruments C2000 Processors  SourceProductBaseCode=TIC2000
  Constant : Constant  Priority=0  OutDataTypeStr=uint8  SampleTime=-1
  Constant1 : Constant  Priority=15  Value=0  OutDataTypeStr=uint8  SampleTime=-1
  Data Store Write : DataStoreWrite  DataStoreName=U1
  Data Store Write1 : DataStoreWrite  DataStoreName=V1
  Data Store Write2 : DataStoreWrite  DataStoreName=W1
  Data Store Write3 : DataStoreWrite  DataStoreName=ATEMP_MCU1
  Data Store Write4 : DataStoreWrite  DataStoreName=ATEMP_MCU2
  Demux : Demux  Outputs=5
  Digital Output : c2833xlib/Digital Output  GPIO_Number=GPIO48~GPIO55  GPIO_Bit0=off  GPIO_BIT0_Toggle=off  GPIO_Bit1=off  GPIO_BIT1_Toggle=off  GPIO_Bit2=off  GPIO_BIT2_Toggle=off  GPIO_Bit3=off  GPIO_BIT3_Toggle=off  GPIO_Bit4=on  GPIO_BIT4_Toggle=off  GPIO_Bit5=off  GPIO_BIT5_Toggle=off  GPIO_Bit6=off  GPIO_BIT6_Toggle=off  GPIO_Bit7=off  GPIO_BIT7_Toggle=off
      settings: SourceProductName=Embedded Coder Support Package for Texas Instruments C2000 Processors  SourceProductBaseCode=TIC2000
  Digital Output1 : c2833xlib/Digital Output  GPIO_Number=GPIO48~GPIO55  GPIO_Bit0=off  GPIO_BIT0_Toggle=off  GPIO_Bit1=off  GPIO_BIT1_Toggle=off  GPIO_Bit2=off  GPIO_BIT2_Toggle=off  GPIO_Bit3=off  GPIO_BIT3_Toggle=off  GPIO_Bit4=on  GPIO_BIT4_Toggle=off  GPIO_Bit5=off  GPIO_BIT5_Toggle=off  GPIO_Bit6=off  GPIO_BIT6_Toggle=off  GPIO_Bit7=off  GPIO_BIT7_Toggle=off
      settings: SourceProductName=Embedded Coder Support Package for Texas Instruments C2000 Processors  SourceProductBaseCode=TIC2000
  Initial Case : Subsystem  TreatAsAtomicUnit=on
  Interrupt_Count : Subsystem  Priority=9  TreatAsAtomicUnit=on
      settings: RTWSystemCode=Inline
  "Main Case " : Subsystem  TreatAsAtomicUnit=on
  "Offset Case " : Subsystem  TreatAsAtomicUnit=on
  Switch Case : SwitchCase  CaseConditions={0,1,2}  ShowDefaultCase=off
  wires:
  ADC/1 -> Demux/1
  Switch Case/2 -> "Offset Case "/Action
  Switch Case/1 -> Initial Case/Action
  Switch Case/3 -> "Main Case "/Action
  Interrupt_Count/1(Out1) -> Switch Case/1
  Constant/1 -> Digital Output/1
  Constant1/1 -> Digital Output1/1
  Demux/4 -> Data Store Write3/1
  Demux/5 -> Data Store Write4/1
  Demux/1 -> Data Store Write/1
  Demux/2 -> Data Store Write1/1
  Demux/3 -> Data Store Write2/1

== system Fuel_Pump_V3_1_20201113_20KHz/NOTE ==
  note: 1kW 燃油泵程序 V1.0
      | 目前已实现了控制板上的全部功能包括：IIC,SCI,PWM,AD2S1210,AD,NTC,PT100,GPIO
      | 对1kW燃油泵电机实现了9,500r/min空载,控制部分代码保存在ram_funs中并使用了Embedd
      | Coder Quick Start对代码进行了优化。
      | 存在问题：
      | 未按照项目计划书对观测变量进行命名
      | 解决电流环PI需要在VVF和停止模式下无法清零
      | AD2S1210启动计划更改在外部而不是中断内部
      | 规定需要的错误保护标志位
      |
      | 1kW燃油泵程序V1.1
      | 之前提到的问题已经解决
      | 修正bug
      | 修正了转速斜坡的给定频率，目前约为2600r/s
      | 修正了转速环积分的初始值错误的问题
      | 目前AD2S1210与IIC温度读取均采用状态机放在定时器中运行
      | 转速计算与位置读取频率分别为1K与20K的固定频率
      | 重写了rampcontrol DMC库中的ramp斜率修改较为复杂，重写
      | 存在问题：
      | 转速上升速度提高后，电机功率相比之前的功率升高【目前无法确定程序的错误问题，把程序回滚到2020_05_20版本后重新修改斜坡给定，功率正常】
      |
      | 1kW燃油泵程序V1.2
      | fuel_pump_new从今天起为薪王
      |
      | 1kW燃油泵程序
      | 修改程序，尝试将运行时间压缩入50us
  note: 1kW 燃油泵程序 V3.1
      | 增加了SMA-SMO滑膜观测器
      | 修正了电流环和转速环的PI逻辑和参数
      | 删除了所有的定点数的计算，缩减程序执行时间
      | 修改了转速计算时的错误，错误的选取了21个控制周期
      | 有框电机中点193，实验电机中点64284
